simulink model "dy3por"  (Simulink 7.5)
settings: Solver=ode45  StartTime=0.0  StopTime=3.56  RelTol=1e-3
settings Model: Creator=Dranik_win  LastModifiedBy=Dranik_win

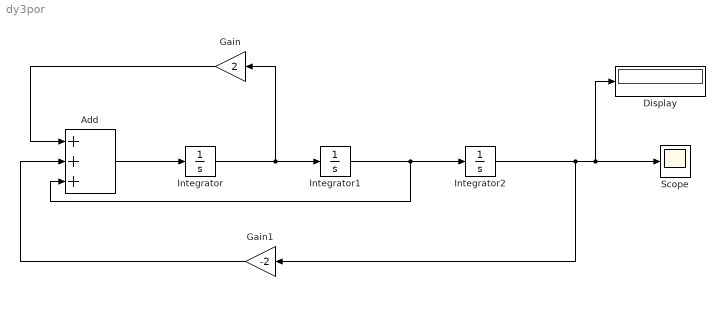
== system dy3por ==
  Add : Sum  Inputs=+++  OutDataType=fixdt(1, 16)  OutScaling=2^-10
  Display : Display
  Gain : Gain  Gain=2  ParameterDataType=fixdt(1, 16)  ParameterScaling=2^0  OutDataType=fixdt(1, 16)  OutScaling=2^0
  Gain1 : Gain  Gain=-2  ParameterDataType=fixdt(1, 16)  ParameterScaling=2^0  OutDataType=fixdt(1, 16)  OutScaling=2^0
  Integrator : Integrator  InitialCondition=3
  Integrator1 : Integrator  InitialCondition=2
  Integrator2 : Integrator  InitialCondition=1
  Scope : Scope
  wires:
  Integrator/1 -> Integrator1/1, Gain/1
  Integrator1/1 -> Integrator2/1, Add/3
  Integrator2/1 -> Gain1/1, Scope/1, Display/1
  Gain/1 -> Add/1
  Add/1 -> Integrator/1
  Gain1/1 -> Add/2
